simulink model "CoVeh_SpdCoord"  (R2016b)
settings: configuration reference "CodeGenConfigSet" (kept outside this file)
settings Model: Creator=Colin  LastModifiedBy=Colin
settings ConfigSetRef: SourceLocation=Base Workspace

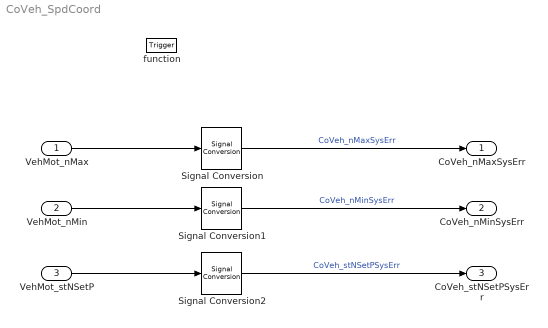
== system CoVeh_SpdCoord ==
  VehMot_nMax : Inport  Tag=rpm  Description=Maximum engine speed for VehMot  OutMin=-12000  OutMax=12000  OutDataTypeStr=EngSpeed_rpm
  VehMot_nMin : Inport  Tag=rpm  Description=Minimum engine speed for VehMot  Port=2  OutMin=-12000  OutMax=12000  OutDataTypeStr=EngSpeed_rpm
  VehMot_stNSetP : Inport  Description=Status of engine speed request after driving assistance coordination  Port=3  OutMin=0  OutMax=255  OutDataTypeStr=State_uint8
  function : TriggerPort  TriggerType=function-call  VariantControl=Variant
  Signal Conversion : SignalConversion  OverrideOpt=off
  Signal Conversion1 : SignalConversion  OverrideOpt=off
  Signal Conversion2 : SignalConversion  OverrideOpt=off
  CoVeh_nMaxSysErr : Outport  Tag=rpm  Description=Maximum speed limitation in case of system errors  OutMin=-12000  OutMax=12000  OutDataTypeStr=EngSpeed_rpm
  CoVeh_nMinSysErr : Outport  Tag=rpm  Description=Minimum speed limitation in case of system errors  Port=2  OutMin=-12000  OutMax=12000  OutDataTypeStr=EngSpeed_rpm
  CoVeh_stNSetPSysErr : Outport  Description=Status word which defines the conversion of the system error speed requirements  Port=3  OutMin=0  OutMax=255  OutDataTypeStr=State_uint8
  wires:
  VehMot_nMax/1 -> Signal Conversion/1
  VehMot_nMin/1 -> Signal Conversion1/1
  VehMot_stNSetP/1 -> Signal Conversion2/1
  Signal Conversion/1 -> CoVeh_nMaxSysErr/1  "CoVeh_nMaxSysErr"
  Signal Conversion1/1 -> CoVeh_nMinSysErr/1  "CoVeh_nMinSysErr"
  Signal Conversion2/1 -> CoVeh_stNSetPSysErr/1  "CoVeh_stNSetPSysErr"
